simulink model "sim_control_speed_distance"  (R2017a)
settings: Solver=VariableStepAuto  StartTime=0.0  StopTime=10.0  RelTol=1e-3
values from neighbouring files (symbols this model uses):
  Coeff_Gd = cell2mat(den)    [control_speed.m]
  Coeff_Gn = cell2mat(num)    [control_speed.m]
  Coeffdd = cell2mat(den)    [control_speed.m]    (also in motor_model.m)
  Coeffnd = cell2mat(num)    [control_speed.m]    (also in motor_model.m)
  Tech = 1/fech    (= 0.00516525128054)    [control_speed.m]    (also in motor_model.m)
libraries: simulink x3
settings Model: Creator=hugo  LastModifiedBy=hugo

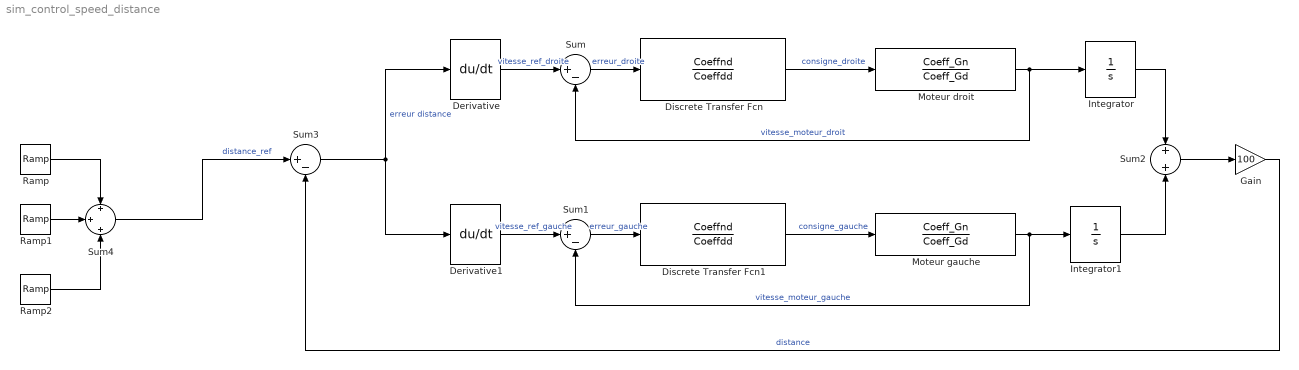
== system sim_control_speed_distance ==
  Derivative : Derivative
  Derivative1 : Derivative
  Discrete Transfer Fcn : DiscreteTransferFcn  Numerator=Coeffnd  Denominator=Coeffdd  SampleTime=Tech
  Discrete Transfer Fcn1 : DiscreteTransferFcn  Numerator=Coeffnd  Denominator=Coeffdd  SampleTime=Tech
  Gain : Gain  Gain=100
  Integrator : Integrator
  Integrator1 : Integrator
  Moteur droit : TransferFcn  Numerator=Coeff_Gn  Denominator=Coeff_Gd
  Moteur gauche : TransferFcn  Numerator=Coeff_Gn  Denominator=Coeff_Gd
  Ramp : simulink/Sources/Ramp  slope=2  start=0  X0=0
  Ramp1 : simulink/Sources/Ramp  slope=-2  start=3  X0=0
  Ramp2 : simulink/Sources/Ramp  slope=-2  start=6  X0=0
  Sum : Sum  Inputs=|+-
  Sum1 : Sum  Inputs=|+-
  Sum2 : Sum  Inputs=+|+
  Sum3 : Sum  Inputs=|+-
  Sum4 : Sum  Inputs=+|+|+
  wires:
  Discrete Transfer Fcn/1 -> Moteur droit/1  "consigne_droite"
  Sum/1 -> Discrete Transfer Fcn/1  "erreur_droite"
  Moteur droit/1 -> Integrator/1, Sum/2  "vitesse_moteur_droit"
  Derivative/1 -> Sum/1  "vitesse_ref_droite"
  Sum1/1 -> Discrete Transfer Fcn1/1  "erreur_gauche"
  Discrete Transfer Fcn1/1 -> Moteur gauche/1  "consigne_gauche"
  Derivative1/1 -> Sum1/1  "vitesse_ref_gauche"
  Moteur gauche/1 -> Integrator1/1, Sum1/2  "vitesse_moteur_gauche"
  Integrator/1 -> Sum2/1
  Integrator1/1 -> Sum2/2
  Sum3/1 -> Derivative/1, Derivative1/1  "erreur distance"
  Ramp/1 -> Sum4/1
  Ramp1/1 -> Sum4/2
  Ramp2/1 -> Sum4/3
  Sum4/1 -> Sum3/1  "distance_ref"
  Sum2/1 -> Gain/1
  Gain/1 -> Sum3/2  "distance"
